simulink model "single_agv_baseline"  (R2025a)
settings: Solver=VariableStepAuto  StartTime=0.0  StopTime=400  RelTol=1e-3
undefined symbols (not defined in the file): Ad, Bd, d_sel, K, p, Ts, x0
libraries: simulink x1
settings Model: Creator=pc  LastModifiedBy=pc

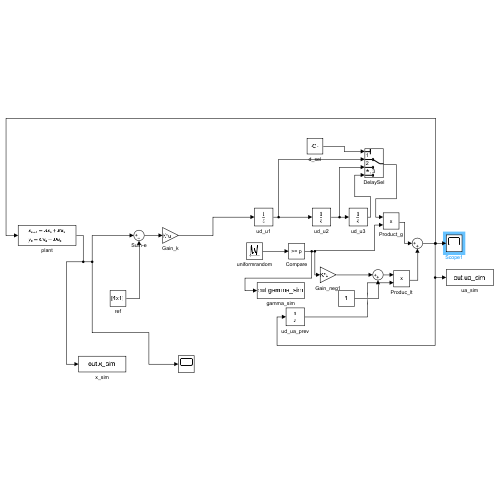
[thumbnail: Simulink's stored preview of the top-level diagram]
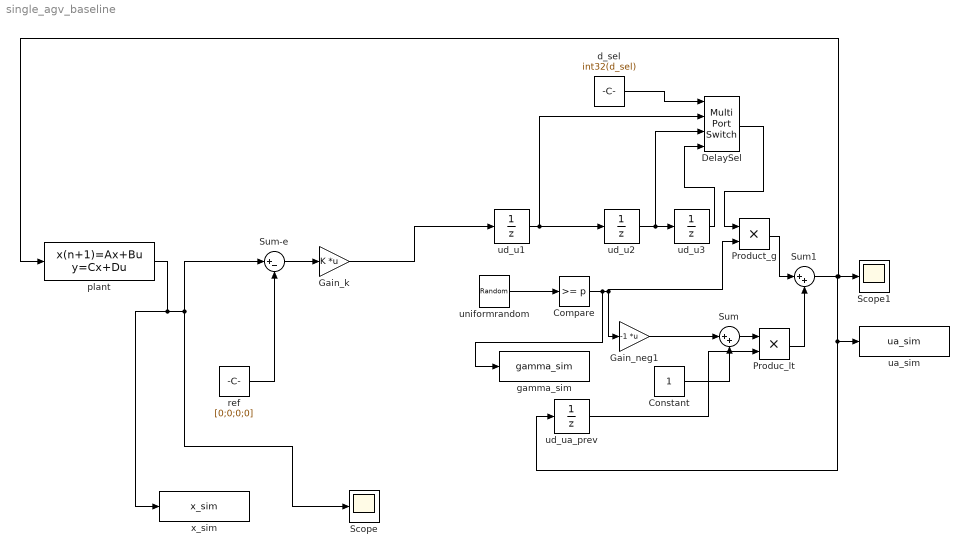
== system single_agv_baseline ==
  "Compare " : simulink/Logic and Bit Operations/Compare To Constant  relop=>=  const=p  OutDataTypeStr=boolean
  Constant : Constant
  DelaySel : MultiPortSwitch  DataPortOrder=Specify indices  DiagnosticForDefault=None  SaturateOnIntegerOverflow=off  InputSameDT=off
  Gain_k : Gain  Gain=K  Multiplication=Matrix(K*u)
  Gain_neg1 : Gain  Gain=-1  Multiplication=Matrix(K*u)
  Produc_lt : Product
  Product_g : Product
  Scope : Scope
      settings: ActiveDisplayYMinimum=-2.3763564372648447  ActiveDisplayYMaximum=2.5351113865945183
  Scope1 : Scope
      settings: ActiveDisplayYMinimum=-0.47859341881740008  ActiveDisplayYMaximum=0.41989771809776977
  Sum : Sum  Inputs=|++
  Sum-e : Sum  Inputs=|+-
  Sum1 : Sum  Inputs=|++
  d_sel : Constant  Value=int32(d_sel)
  gamma_sim : ToWorkspace  VariableName=gamma_sim  SaveFormat=Timeseries  SampleTime=-1
  plant : DiscreteStateSpace  A=Ad  B=Bd  C=eye(4)  D=zeros(4,2)  InitialCondition=x0  SampleTime=Ts
  ref : Constant  Value=[0;0;0;0]
  ua_sim : ToWorkspace  VariableName=ua_sim  SaveFormat=Timeseries  SampleTime=-1
  ud_u1 : UnitDelay  InitialCondition=[0;0]  SampleTime=Ts  HasFrameUpgradeWarning=on
  ud_u2 : UnitDelay  InitialCondition=[0;0]  SampleTime=Ts  HasFrameUpgradeWarning=on
  ud_u3 : UnitDelay  InitialCondition=[0;0]  SampleTime=Ts  HasFrameUpgradeWarning=on
  ud_ua_prev : UnitDelay  InitialCondition=[0;0]  SampleTime=Ts  HasFrameUpgradeWarning=on
  uniformrandom : UniformRandomNumber  Minimum=0  SampleTime=Ts
  x_sim : ToWorkspace  VariableName=x_sim  SaveFormat=Timeseries  SampleTime=-1
  wires:
  plant/1 -> x_sim/1, Scope/1, Sum-e/1
  Sum-e/1 -> Gain_k/1
  ref/1 -> Sum-e/2
  Gain_k/1 -> ud_u1/1
  ud_u1/1 -> ud_u2/1, DelaySel/2
  ud_u2/1 -> DelaySel/3, ud_u3/1
  uniformrandom/1 -> "Compare "/1
  "Compare "/1 -> gamma_sim/1, Product_g/2, Gain_neg1/1
  Gain_neg1/1 -> Sum/1
  Constant/1 -> Sum/2
  Sum/1 -> Produc_lt/1
  ud_ua_prev/1 -> Produc_lt/2
  Product_g/1 -> Sum1/1
  Produc_lt/1 -> Sum1/2
  Sum1/1 -> Scope1/1, plant/1, ua_sim/1, ud_ua_prev/1
  DelaySel/1 -> Product_g/1
  d_sel/1 -> DelaySel/1
  ud_u3/1 -> DelaySel/4
